simulink model "test_fmu"  (R2022a)
settings: Solver=FixedStepAuto  StartTime=0.0  StopTime=10.0  RelTol=1e-3
settings Model: Creator=lordx  LastModifiedBy=lordx
settings RTWCC: Description=FMU based on GRT (Functional Mock-up Unit)  SystemTargetFile=grtfmi.tlc  GenerateMakefile=off  TemplateMakefile=none  GenerateReport=on  RetainRTWFile=on
settings CodeAppCC: ForceParamTrailComments=on  StateflowObjectComments=on  MATLABSourceComments=on
settings STFCustomTargetCC: TargetLangStandard=C99 (ISO)  CombineOutputUpdateFcns=on  GRTInterface=off  SystemTargetFile=grtfmi.tlc
settings GRTTargetCC: ParMdlRefBuildCompliant=off  CompOptLevelCompliant=off  ConcurrentExecutionCompliant=off  MatFileLogging=off  CPPClassGenCompliant=off  UseToolchainInfoCompliant=off  RTWCAPISignals=on  RTWCAPIParams=on  RTWCAPIStates=on  RTWCAPIRootIO=on

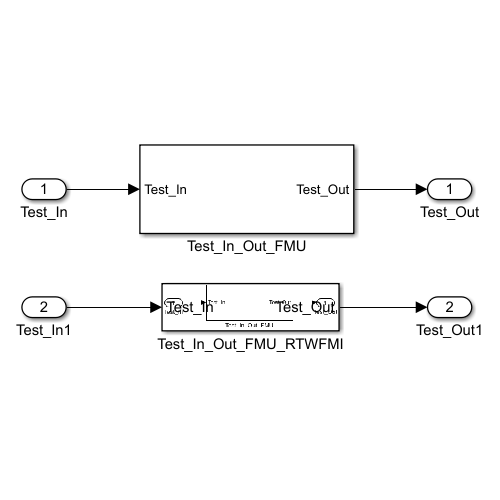
[thumbnail: Simulink's stored preview of the top-level diagram]
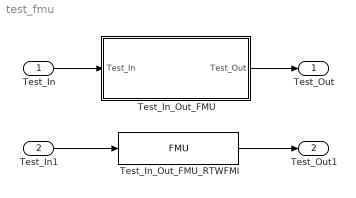
== system test_fmu ==
  Test_In : Inport
  Test_In1 : Inport  Port=2
  Test_In_Out_FMU : Subsystem
  Test_In_Out_FMU_RTWFMI : FMU  FMUName=test_fmu.fmu  FMUDebugLogging=on  FMUMode=CoSimulation  Parameters_Gain_Gain=10  mask(test_fmu [Co-Simulation, v3.0]){}
      mask Display:
      | if (exist([Simulink.fileGenControl('get','CacheFolder') '\slprj\_fmu\99735fa8c935bada74a203303a60adf9\test_fmu\model.png'],'file'))
      |     image([Simulink.fileGenControl('get','CacheFolder') '\slprj\_fmu\99735fa8c935bada74a203303a60adf9\test_fmu\model.png']);
      | else
      |     disp('test_fmu [Co-Simulation, v3.0]');
      | end
      | port_label('output',1,'Test_Out');
      | port_label('input',1,'Test_In');
  Test_Out : Outport
  Test_Out1 : Outport  Port=2
  wires:
  Test_In/1 -> Test_In_Out_FMU/1(Test_In)
  Test_In_Out_FMU/1(Test_Out) -> Test_Out/1
  Test_In1/1 -> Test_In_Out_FMU_RTWFMI/1
  Test_In_Out_FMU_RTWFMI/1 -> Test_Out1/1

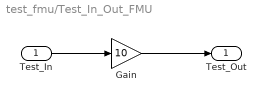
== system test_fmu/Test_In_Out_FMU ==
  Test_In : Inport
  Gain : Gain  Gain=10
  Test_Out : Outport
  wires:
  Test_In/1 -> Gain/1
  Gain/1 -> Test_Out/1
